simulink model "untitled - Copy"  (R2020b)
settings: Solver=VariableStepAuto  StartTime=0.0  StopTime=10.0  RelTol=1e-3
model workspace (MAT data in the model file):
  kE = Simulink.Parameter
  kE.DataType = 'auto'
  kE.Dimensions = [0 0]
values from neighbouring files (symbols this model uses):
  kc = 125    [params.m]
  kE = 1000    [params.m]
  kp = 500    [params.m]
  Tc = 300    [params.m]
  Tp = 60    [params.m]
settings Model: Creator=olaru  LastModifiedBy=olaru

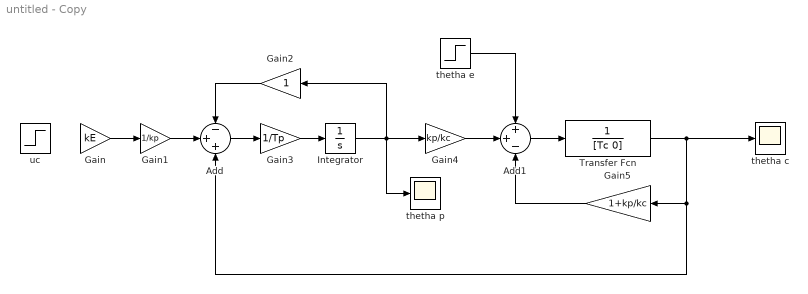
== system untitled - Copy ==
  Add : Sum  Inputs=-++
  Add1 : Sum  Inputs=++-
  Gain : Gain  Gain=kE
  Gain1 : Gain  Gain=1/kp
  Gain2 : Gain
  Gain3 : Gain  Gain=1/Tp
  Gain4 : Gain  Gain=kp/kc
  Gain5 : Gain  Gain=1+kp/kc
  Integrator : Integrator
  Transfer Fcn : TransferFcn  Denominator=[Tc 0]
  thetha c : Scope
  thetha e : Step  SampleTime=0
  thetha p : Scope
  uc : Step  SampleTime=0
  wires:
  Gain/1 -> Gain1/1
  Gain1/1 -> Add/2
  Gain2/1 -> Add/1
  Add/1 -> Gain3/1
  Gain3/1 -> Integrator/1
  Integrator/1 -> thetha p/1, Gain4/1, Gain2/1
  Gain4/1 -> Add1/2
  Add1/1 -> Transfer Fcn/1
  Gain5/1 -> Add1/3
  Transfer Fcn/1 -> thetha c/1, Add/3, Gain5/1
  thetha e/1 -> Add1/1
